simulink model "gm_sampleModel1775_4_sub"  (R2023a)
settings: Solver=VariableStepAuto  StartTime=0.0  StopTime=10.0  RelTol=1e-3
libraries: simulink x4
settings Model: Creator=user1  LastModifiedBy=user1
settings OptimizationCC: BlockReduction=off  ConditionallyExecuteInputs=off
settings DebuggingCC: InheritedTsInSrcMsg=none

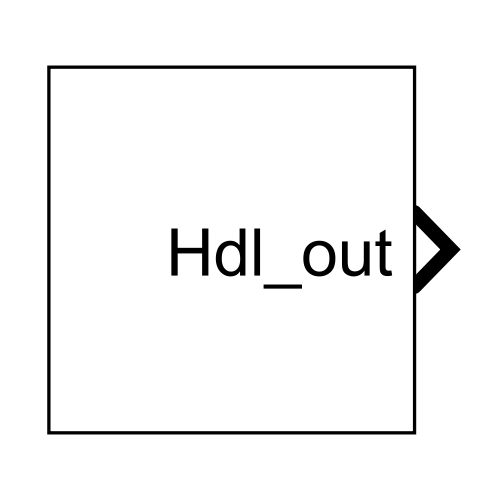
[thumbnail: Simulink's stored preview of the top-level diagram]
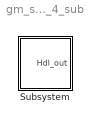
== system gm_sampleModel1775_4_sub ==
  Subsystem : Subsystem

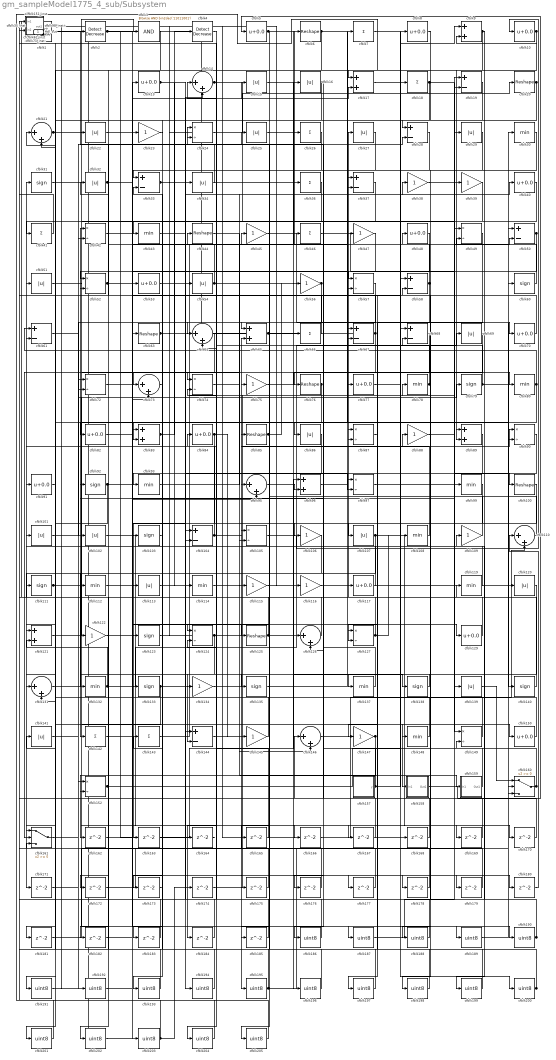
== system gm_sampleModel1775_4_sub/Subsystem ==
  cfblk1 : simulink/Logic and Bit Operations/Detect Decrease  vinit=0.0  OutDataTypeStr=uint8
      settings: LibrarySourceBlock=|
      | hdlsllib/Logic and Bit
      | Operations/Detect
      | Decrease
  cfblk{5,8,10,13,40,48,53,70,77,82,84,91,117,129,150} (15 alike) : Bias  Bias=0.0  SaturateOnIntegerOverflow=off
  cfblk{6,20,44,63,76,85,100,125} (8 alike) : Reshape
  cfblk{15..16,22,25,27,29,32,34,51,54,69,86,101..102,107,113,120,139,141} (19 alike) : Abs  OutDataTypeStr=uint8  SaturateOnIntegerOverflow=off
  cfblk{31,60,79,92,103,111,123,133,135,138,140} (11 alike) : Signum
  cfblk{19,28,33,37,50,58,61,67..68,104,144} (11 alike) : Sum  Inputs=+-  OutDataTypeStr=uint8
  cfblk{24,42,49,52,57,72,74,87,90,97,105,124,127,149,152} (15 alike) : Product  Inputs=*/  OutDataTypeStr=uint8  RndMeth=Zero  SaturateOnIntegerOverflow=on
  cfblk{23,38..39,45,47,56,75,88,106,109,115..116,122,134,145,147} (16 alike) : Gain  OutDataTypeStr=uint8
  cfblk{30,43,78,80,93,99,108,112,114,119,132,137,148} (13 alike) : MinMax  OutDataTypeStr=uint8
  cfblk{14,21,64,73,95,110,126,131,146} (9 alike) : Sum  Inputs=|++  OutDataTypeStr=uint8
  cfblk118_inst : Subsystem
  cfblk11_inst : Subsystem
  cfblk{9,17,65,83,89,96,121} (7 alike) : Sum  OutDataTypeStr=uint8
  cfblk128_inst : Subsystem
  cfblk130_inst : Subsystem
  cfblk136_inst : Subsystem
  cfblk{7,18,26,36,41,46,66,142..143} (9 alike) : Sum  Inputs=+  OutDataTypeStr=uint8
  cfblk151_inst : Subsystem
  cfblk157 : Subsystem  mask(Counter Limited){uplimit=double(7), tsamp=double(-1)}
      mask prompts: uplimit "Simulink:masks:UpperLimit_MP"; tsamp "Simulink:masks:SampleTime_MP"
      mask help: Simulink:masks:CounterLimited_MD
      mask init:
      | nbits = double(8);
      | tsamp = double(-1);
      | uplimit = double(7);
  cfblk158 : Subsystem
  cfblk159 : Subsystem
  cfblk160 : Switch  OutDataTypeStr=uint8  SaturateOnIntegerOverflow=off  InputSameDT=off
  cfblk161 : Switch  OutDataTypeStr=uint8  SaturateOnIntegerOverflow=off  InputSameDT=off
  cfblk{162..185} (24 alike) : Delay  SampleTime=1
  cfblk{186..205} (20 alike) : DataTypeConversion  OutDataTypeStr=uint8  SaturateOnIntegerOverflow=off  RndMeth=Floor
  cfblk2 : simulink/Logic and Bit Operations/Detect Decrease  vinit=0.0  OutDataTypeStr=uint8
      settings: LibrarySourceBlock=|
      | hdlsllib/Logic and Bit
      | Operations/Detect
      | Decrease
  cfblk3 : simulink/Logic and Bit Operations/Bitwise Operator  logicop=AND  UseBitMask=on  BitMask=bin2dec('11011001')  BitMaskRealWorld=Stored Integer
      settings: LibrarySourceBlock=|
      | hdlsllib/Logic and Bit
      | Operations/Bitwise
      | Operator
  cfblk35_inst : Subsystem
  cfblk4 : simulink/Logic and Bit Operations/Detect Decrease  vinit=0.0  OutDataTypeStr=uint8
      settings: LibrarySourceBlock=|
      | hdlsllib/Logic and Bit
      | Operations/Detect
      | Decrease
  cfblk62_inst : Subsystem
  cfblk71_inst : Subsystem
  cfblk98_inst : Subsystem
  Hdl_out : Outport  OutDataTypeStr=uint8  SampleTime=1
  wires:
  cfblk1/1 -> cfblk83/2, cfblk3/1, cfblk187/1
  cfblk10/1 -> cfblk9/2, cfblk89/2
  cfblk100/1 -> cfblk163/1
  cfblk101/1 -> cfblk166/1
  cfblk102/1 -> cfblk129/1
  cfblk103/1 -> cfblk193/1
  cfblk104/1 -> cfblk31/1, cfblk88/1
  cfblk105/1 -> cfblk10/1
  cfblk106/1 -> cfblk142/1
  cfblk107/1 -> cfblk171/1, cfblk170/1
  cfblk108/1 -> cfblk65/2
  cfblk109/1 -> cfblk44/1
  cfblk11_inst/1(out1) -> cfblk66/1
  cfblk110/1 -> cfblk45/1
  cfblk111/1 -> cfblk191/1, cfblk158/1(In1)
  cfblk112/1 -> cfblk195/1
  cfblk113/1 -> cfblk6/1
  cfblk114/1 -> cfblk75/1
  cfblk115/1 -> cfblk90/1
  cfblk116/1 -> cfblk27/1
  cfblk117/1 -> cfblk61/2
  cfblk118_inst/1(out1) -> cfblk26/1
  cfblk119/1 -> cfblk67/2
  cfblk120/1 -> cfblk144/2
  cfblk121/1 -> cfblk79/1
  cfblk122/1 -> cfblk184/1
  cfblk123/1 -> cfblk16/1
  cfblk124/1 -> cfblk29/1, cfblk202/1
  cfblk125/1 -> cfblk151_inst/1(in1), cfblk123/1
  cfblk126/1 -> cfblk21/1
  cfblk127/1 -> cfblk98_inst/1(in1), cfblk108/1
  cfblk128_inst/1(out1) -> cfblk203/1
  cfblk129/1 -> cfblk91/1
  cfblk13/1 -> cfblk54/1, cfblk34/1
  cfblk130_inst/1(out1) -> cfblk36/1
  cfblk131/1 -> cfblk42/1
  cfblk132/1 -> cfblk69/1, cfblk21/2
  cfblk133/1 -> cfblk37/1, cfblk181/1
  cfblk134/1 -> cfblk67/1
  cfblk135/1 -> cfblk7/1
  cfblk136_inst/1(out1) -> cfblk192/1
  cfblk137/1 -> cfblk101/1
  cfblk138/1 -> cfblk137/1
  cfblk139/1 -> cfblk160/1
  cfblk14/1 -> cfblk204/1, cfblk116/1
  cfblk140/1 -> cfblk62_inst/2(in2)
  cfblk141/1 -> cfblk72/1
  cfblk142/1 -> cfblk194/1
  cfblk143/1 -> cfblk78/1
  cfblk144/1 -> cfblk150/1
  cfblk145/1 -> cfblk130_inst/1(in1)
  cfblk146/1 -> cfblk110/2
  cfblk147/1 -> cfblk162/1, cfblk152/2
  cfblk148/1 -> cfblk24/1
  cfblk149/1 -> cfblk117/1
  cfblk15/1 -> cfblk178/1
  cfblk150/1 -> cfblk95/1
  cfblk151_inst/1(out1) -> cfblk53/1, cfblk23/1
  cfblk152/1 -> cfblk14/2, cfblk122/1, cfblk18/1
  cfblk157/1(y) -> cfblk9/1, cfblk24/2
  cfblk158/1(Out1) -> cfblk5/1
  cfblk159/1(Out1) -> cfblk149/2
  cfblk16/1 -> cfblk161/1, cfblk106/1
  cfblk160/1 -> cfblk92/1, cfblk119/1
  cfblk161/1 -> cfblk28/2
  cfblk162/1 -> cfblk97/1
  cfblk163/1 -> cfblk96/1
  cfblk164/1 -> cfblk1/1
  cfblk165/1 -> cfblk74/2
  cfblk166/1 -> cfblk49/1
  cfblk167/1 -> cfblk126/2
  cfblk168/1 -> cfblk57/2
  cfblk169/1 -> cfblk146/1
  cfblk17/1 -> cfblk200/1
  cfblk170/1 -> cfblk71_inst/1(in1)
  cfblk171/1 -> cfblk42/2
  cfblk172/1 -> cfblk160/2
  cfblk173/1 -> cfblk33/2
  cfblk174/1 -> cfblk19/2
  cfblk175/1 -> cfblk131/2
  cfblk176/1 -> cfblk62_inst/1(in1)
  cfblk177/1 -> cfblk124/2
  cfblk178/1 -> cfblk152/1
  cfblk179/1 -> cfblk105/1
  cfblk18/1 -> cfblk100/1, cfblk52/1, cfblk183/1
  cfblk180/1 -> cfblk110/1
  cfblk181/1 -> cfblk50/1
  cfblk182/1 -> cfblk95/2
  cfblk183/1 -> cfblk121/2
  cfblk184/1 -> cfblk144/1
  cfblk185/1 -> cfblk35_inst/2(in2)
  cfblk186/1 -> cfblk141/1
  cfblk187/1 -> cfblk99/1
  cfblk188/1 -> cfblk84/1
  cfblk189/1 -> cfblk30/1
  cfblk19/1 -> cfblk43/1
  cfblk190/1 -> cfblk68/2, cfblk11_inst/1(in1), cfblk109/1
  cfblk191/1 -> cfblk77/1
  cfblk192/1 -> cfblk63/1
  cfblk193/1 -> cfblk136_inst/1(in1)
  cfblk194/1 -> cfblk136_inst/2(in2)
  cfblk195/1 -> cfblk160/3, cfblk130_inst/2(in2), cfblk143/1
  cfblk196/1 -> cfblk112/1
  cfblk197/1 -> cfblk85/1
  cfblk198/1 -> cfblk87/1
  cfblk199/1 -> cfblk87/2
  cfblk2/1 -> cfblk189/1, cfblk127/2
  cfblk20/1 -> cfblk82/1, cfblk125/1
  cfblk200/1 -> cfblk161/3, cfblk118_inst/2(in2)
  cfblk201/1 -> cfblk17/1
  cfblk202/1 -> cfblk17/2
  cfblk203/1 -> cfblk151_inst/2(in2), cfblk174/1
  cfblk204/1 -> cfblk128_inst/1(in1)
  cfblk205/1 -> cfblk128_inst/2(in2)
  cfblk21/1 -> cfblk73/2, cfblk104/1
  cfblk22/1 -> cfblk15/1
  cfblk23/1 -> cfblk103/1
  cfblk24/1 -> cfblk8/1
  cfblk25/1 -> cfblk20/1
  cfblk26/1 -> cfblk164/1
  cfblk27/1 -> cfblk33/1
  cfblk28/1 -> cfblk165/1
  cfblk29/1 -> cfblk76/1
  cfblk3/1 -> cfblk131/1
  cfblk30/1 -> cfblk188/1
  cfblk31/1 -> cfblk139/1
  cfblk32/1 -> cfblk104/2, cfblk179/1
  cfblk33/1 -> cfblk37/2, cfblk169/1, cfblk114/1
  cfblk34/1 -> cfblk2/1
  cfblk35_inst/1(out1) -> cfblk120/1
  cfblk36/1 -> cfblk41/1
  cfblk37/1 -> cfblk135/1
  cfblk38/1 -> cfblk19/1
  cfblk39/1 -> cfblk176/1
  cfblk4/1 -> cfblk64/1
  cfblk40/1 -> cfblk124/1
  cfblk41/1 -> cfblk118_inst/1(in1)
  cfblk42/1 -> cfblk86/1
  cfblk43/1 -> cfblk97/2
  cfblk44/1 -> cfblk159/1(In1)
  cfblk45/1 -> cfblk140/1
  cfblk46/1 -> cfblk149/1
  cfblk47/1 -> cfblk182/1
  cfblk48/1 -> cfblk74/1
  cfblk49/1 -> cfblk147/1
  cfblk5/1 -> cfblk65/1, cfblk177/1
  cfblk50/1 -> cfblk49/2, cfblk185/1
  cfblk51/1 -> cfblk115/1
  cfblk52/1 -> cfblk57/1, cfblk47/1
  cfblk53/1 -> cfblk90/2
  cfblk54/1 -> cfblk70/1, cfblk32/1, cfblk196/1
  cfblk56/1 -> cfblk73/1, cfblk64/2
  cfblk57/1 -> cfblk72/2
  cfblk58/1 -> cfblk14/1, cfblk127/1
  cfblk6/1 -> cfblk89/1, cfblk132/1
  cfblk60/1 -> cfblk48/1
  cfblk61/1 -> cfblk102/1
  cfblk62_inst/1(out1) -> cfblk35_inst/1(in1)
  cfblk63/1 -> cfblk175/1, cfblk148/1
  cfblk64/1 -> cfblk172/1
  cfblk65/1 -> cfblk138/1, cfblk167/1
  cfblk66/1 -> cfblk22/1
  cfblk67/1 -> cfblk98_inst/2(in2), cfblk161/2, Hdl_out/1
  cfblk68/1 -> cfblk83/1
  cfblk69/1 -> cfblk198/1
  cfblk7/1 -> cfblk68/1
  cfblk70/1 -> cfblk71_inst/2(in2)
  cfblk71_inst/1(out1) -> cfblk126/1
  cfblk72/1 -> cfblk13/1
  cfblk73/1 -> cfblk93/1
  cfblk74/1 -> cfblk146/2
  cfblk75/1 -> cfblk80/1
  cfblk76/1 -> cfblk205/1, cfblk111/1
  cfblk77/1 -> cfblk190/1
  cfblk78/1 -> cfblk58/2, cfblk11_inst/2(in2), cfblk46/1
  cfblk79/1 -> cfblk60/1, cfblk52/2
  cfblk8/1 -> cfblk28/1
  cfblk80/1 -> cfblk61/1, cfblk134/1
  cfblk82/1 -> cfblk180/1
  cfblk83/1 -> cfblk173/1, cfblk4/1
  cfblk84/1 -> cfblk113/1, cfblk145/1
  cfblk85/1 -> cfblk25/1, cfblk56/1
  cfblk86/1 -> cfblk105/2
  cfblk87/1 -> cfblk197/1
  cfblk88/1 -> cfblk39/1
  cfblk89/1 -> cfblk133/1
  cfblk9/1 -> cfblk199/1, cfblk121/1
  cfblk90/1 -> cfblk107/1
  cfblk91/1 -> cfblk51/1
  cfblk92/1 -> cfblk58/1, cfblk201/1
  cfblk93/1 -> cfblk40/1
  cfblk95/1 -> cfblk96/2
  cfblk96/1 -> cfblk38/1
  cfblk97/1 -> cfblk50/2
  cfblk98_inst/1(out1) -> cfblk168/1
  cfblk99/1 -> cfblk186/1

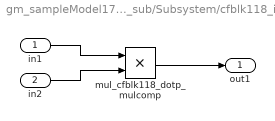
== system gm_sampleModel1775_4_sub/Subsystem/cfblk118_inst ==
  in1 : Inport  OutDataTypeStr=uint8  SampleTime=1
  in2 : Inport  Port=2  OutDataTypeStr=uint8  SampleTime=1
  mul_cfblk118_dotp_mulcomp : Product  Inputs=**  OutDataTypeStr=uint8  SampleTime=1
  out1 : Outport  OutDataTypeStr=uint8  SampleTime=1
  wires:
  in1/1 -> mul_cfblk118_dotp_mulcomp/1
  in2/1 -> mul_cfblk118_dotp_mulcomp/2
  mul_cfblk118_dotp_mulcomp/1 -> out1/1

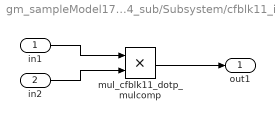
== system gm_sampleModel1775_4_sub/Subsystem/cfblk11_inst ==
  in1 : Inport  OutDataTypeStr=uint8  SampleTime=1
  in2 : Inport  Port=2  OutDataTypeStr=uint8  SampleTime=1
  mul_cfblk11_dotp_mulcomp : Product  Inputs=**  OutDataTypeStr=uint8  SampleTime=1
  out1 : Outport  OutDataTypeStr=uint8  SampleTime=1
  wires:
  in1/1 -> mul_cfblk11_dotp_mulcomp/1
  in2/1 -> mul_cfblk11_dotp_mulcomp/2
  mul_cfblk11_dotp_mulcomp/1 -> out1/1

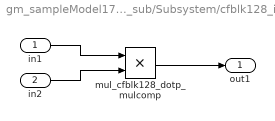
== system gm_sampleModel1775_4_sub/Subsystem/cfblk128_inst ==
  in1 : Inport  OutDataTypeStr=uint8  SampleTime=1
  in2 : Inport  Port=2  OutDataTypeStr=uint8  SampleTime=1
  mul_cfblk128_dotp_mulcomp : Product  Inputs=**  OutDataTypeStr=uint8  SampleTime=1
  out1 : Outport  OutDataTypeStr=uint8  SampleTime=1
  wires:
  in1/1 -> mul_cfblk128_dotp_mulcomp/1
  in2/1 -> mul_cfblk128_dotp_mulcomp/2
  mul_cfblk128_dotp_mulcomp/1 -> out1/1

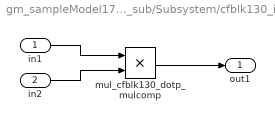
== system gm_sampleModel1775_4_sub/Subsystem/cfblk130_inst ==
  in1 : Inport  OutDataTypeStr=uint8  SampleTime=1
  in2 : Inport  Port=2  OutDataTypeStr=uint8  SampleTime=1
  mul_cfblk130_dotp_mulcomp : Product  Inputs=**  OutDataTypeStr=uint8  SampleTime=1
  out1 : Outport  OutDataTypeStr=uint8  SampleTime=1
  wires:
  in1/1 -> mul_cfblk130_dotp_mulcomp/1
  in2/1 -> mul_cfblk130_dotp_mulcomp/2
  mul_cfblk130_dotp_mulcomp/1 -> out1/1

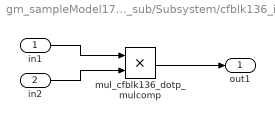
== system gm_sampleModel1775_4_sub/Subsystem/cfblk136_inst ==
  in1 : Inport  OutDataTypeStr=uint8  SampleTime=1
  in2 : Inport  Port=2  OutDataTypeStr=uint8  SampleTime=1
  mul_cfblk136_dotp_mulcomp : Product  Inputs=**  OutDataTypeStr=uint8  SampleTime=1
  out1 : Outport  OutDataTypeStr=uint8  SampleTime=1
  wires:
  in1/1 -> mul_cfblk136_dotp_mulcomp/1
  in2/1 -> mul_cfblk136_dotp_mulcomp/2
  mul_cfblk136_dotp_mulcomp/1 -> out1/1

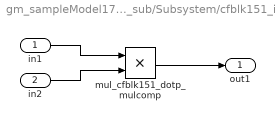
== system gm_sampleModel1775_4_sub/Subsystem/cfblk151_inst ==
  in1 : Inport  OutDataTypeStr=uint8  SampleTime=1
  in2 : Inport  Port=2  OutDataTypeStr=uint8  SampleTime=1
  mul_cfblk151_dotp_mulcomp : Product  Inputs=**  OutDataTypeStr=uint8  SampleTime=1
  out1 : Outport  OutDataTypeStr=uint8  SampleTime=1
  wires:
  in1/1 -> mul_cfblk151_dotp_mulcomp/1
  in2/1 -> mul_cfblk151_dotp_mulcomp/2
  mul_cfblk151_dotp_mulcomp/1 -> out1/1

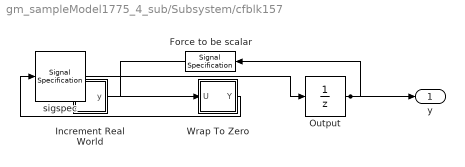
== system gm_sampleModel1775_4_sub/Subsystem/cfblk157 ==
  Force to be scalar : SignalSpecification  DisableCoverage=on  Dimensions=1
  Increment Real World : Subsystem  mask(Real World Value Increment){}
      mask help: Simulink:masks:RealWorldValueIncrement_MD
      mask Display: disp('V++')
  Output : UnitDelay  InitialCondition=0.0  SampleTime=tsamp  HasFrameUpgradeWarning=on
  Wrap To Zero : Subsystem  mask(Wrap To Zero){Threshold=double(7)}
      mask prompts: Threshold "Simulink:masks:Threshold_MP"
      mask help: Simulink:masks:WrapToZero_MD
  sigspec : SignalSpecification  OutDataTypeStr=uint8  Dimensions=1
  y : Outport  SampleTime=1
  wires:
  Force to be scalar/1 -> Increment Real World/1(u)
  Increment Real World/1(y) -> Wrap To Zero/1(U)
  Output/1 -> Force to be scalar/1, y/1
  Wrap To Zero/1(Y) -> sigspec/1
  sigspec/1 -> Output/1

== system gm_sampleModel1775_4_sub/Subsystem/cfblk158 ==
  In1 : Inport  OutDataTypeStr=uint8  PortDimensions=1  SampleTime=1
  Out1 : Outport  SampleTime=1
  wires:
  In1/1 -> Out1/1

== system gm_sampleModel1775_4_sub/Subsystem/cfblk159 ==
  In1 : Inport  OutDataTypeStr=uint8  PortDimensions=1  SampleTime=1
  Out1 : Outport  SampleTime=1
  wires:
  In1/1 -> Out1/1

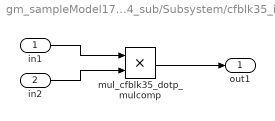
== system gm_sampleModel1775_4_sub/Subsystem/cfblk35_inst ==
  in1 : Inport  OutDataTypeStr=uint8  SampleTime=1
  in2 : Inport  Port=2  OutDataTypeStr=uint8  SampleTime=1
  mul_cfblk35_dotp_mulcomp : Product  Inputs=**  OutDataTypeStr=uint8  SampleTime=1
  out1 : Outport  OutDataTypeStr=uint8  SampleTime=1
  wires:
  in1/1 -> mul_cfblk35_dotp_mulcomp/1
  in2/1 -> mul_cfblk35_dotp_mulcomp/2
  mul_cfblk35_dotp_mulcomp/1 -> out1/1

== system gm_sampleModel1775_4_sub/Subsystem/cfblk62_inst ==
  in1 : Inport  OutDataTypeStr=uint8  SampleTime=1
  in2 : Inport  Port=2  OutDataTypeStr=uint8  SampleTime=1
  mul_cfblk62_dotp_mulcomp : Product  Inputs=**  OutDataTypeStr=uint8  SampleTime=1
  out1 : Outport  OutDataTypeStr=uint8  SampleTime=1
  wires:
  in1/1 -> mul_cfblk62_dotp_mulcomp/1
  in2/1 -> mul_cfblk62_dotp_mulcomp/2
  mul_cfblk62_dotp_mulcomp/1 -> out1/1

== system gm_sampleModel1775_4_sub/Subsystem/cfblk71_inst ==
  in1 : Inport  OutDataTypeStr=uint8  SampleTime=1
  in2 : Inport  Port=2  OutDataTypeStr=uint8  SampleTime=1
  mul_cfblk71_dotp_mulcomp : Product  Inputs=**  OutDataTypeStr=uint8  SampleTime=1
  out1 : Outport  OutDataTypeStr=uint8  SampleTime=1
  wires:
  in1/1 -> mul_cfblk71_dotp_mulcomp/1
  in2/1 -> mul_cfblk71_dotp_mulcomp/2
  mul_cfblk71_dotp_mulcomp/1 -> out1/1

== system gm_sampleModel1775_4_sub/Subsystem/cfblk98_inst ==
  in1 : Inport  OutDataTypeStr=uint8  SampleTime=1
  in2 : Inport  Port=2  OutDataTypeStr=uint8  SampleTime=1
  mul_cfblk98_dotp_mulcomp : Product  Inputs=**  OutDataTypeStr=uint8  SampleTime=1
  out1 : Outport  OutDataTypeStr=uint8  SampleTime=1
  wires:
  in1/1 -> mul_cfblk98_dotp_mulcomp/1
  in2/1 -> mul_cfblk98_dotp_mulcomp/2
  mul_cfblk98_dotp_mulcomp/1 -> out1/1

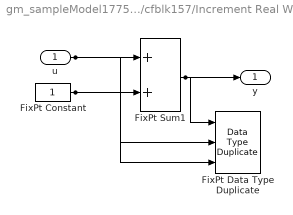
== system gm_sampleModel1775_4_sub/Subsystem/cfblk157/Increment Real World ==
  u : Inport  OutDataTypeStr=uint8  SampleTime=1
  FixPt Constant : Constant  DisableCoverage=on  OutDataTypeStr=Inherit: Inherit via back propagation  SampleTime=-1
  FixPt Data Type Duplicate : DataTypeDuplicate  DisableCoverage=on  NumInputPorts=3
  FixPt Sum1 : Sum  InputSameDT=on  OutDataTypeStr=Inherit: Inherit via back propagation  LockScale=on
  y : Outport  SampleTime=1
  wires:
  u/1 -> FixPt Sum1/1, FixPt Data Type Duplicate/2
  FixPt Constant/1 -> FixPt Sum1/2, FixPt Data Type Duplicate/3
  FixPt Sum1/1 -> FixPt Data Type Duplicate/1, y/1

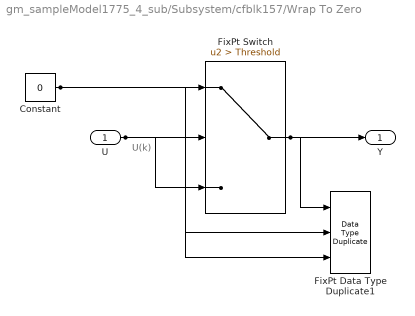
== system gm_sampleModel1775_4_sub/Subsystem/cfblk157/Wrap To Zero ==
  note: U(k)
  U : Inport  OutDataTypeStr=uint8  SampleTime=1
  Constant : Constant  DisableCoverage=on  Value=0  OutDataTypeStr=Inherit: Inherit via back propagation  SampleTime=-1
  FixPt Data Type Duplicate1 : DataTypeDuplicate  DisableCoverage=on  NumInputPorts=3
  FixPt Switch : Switch  Criteria=u2 > Threshold  Threshold=Threshold  OutDataTypeStr=Inherit: Inherit via back propagation  ZeroCross=off  SaturateOnIntegerOverflow=off  InputSameDT=off
  Y : Outport  SampleTime=1
  wires:
  U/1 -> FixPt Switch/3, FixPt Switch/2, FixPt Data Type Duplicate1/2
  Constant/1 -> FixPt Switch/1, FixPt Data Type Duplicate1/3
  FixPt Switch/1 -> FixPt Data Type Duplicate1/1, Y/1
